simulink model "pfb_fir"  (Simulink 7.0)
settings: Solver=FixedStepDiscrete  SolverMode=SingleTasking  StartTime=0.0  StopTime=10.0  RelTol=1e-3
undefined symbols (not defined in the file): pfb_coefs
libraries: xbsIndex_r4 x385
(part 9 of 27)

== system pfb_fir/fir_2/fir_tap_2 ==
  data_in : Inport  OutDataType=sfix(16)  OutScaling=2^0
  sum_in : Inport  Port=2  OutDataType=sfix(16)  OutScaling=2^0
  sync_in : Inport  Port=3  OutDataType=sfix(16)  OutScaling=2^0
  fir_coef : Subsystem  mask(FIR Filter Coefficient Generator){coef=[-0.000375660323525046;-0.00112528207646786;-0.00187263770065757;-0.00261772609063303;-0.00336054616203061;-0.00410109685156988;-0.00483937711704019;-0.00557538593728603;-0.00630912231219222;-0.00704058526266978;-0.00776977383064064;-0.00849668707902262;-0.00922132409171369;-0.00994368397357705;-0.0106637658504249;-0.0113815688690025;-0.0120970921969721;-0.0128103350228962;-0.0135212965562215;-0.0142299760272615;-0.0149363726871797;-0.0156404858079725;-0.0163423146824514;-0.0170418586242254;-0.0177391169676835;-0.0184340890679761;-0.0191267743009973;-0.0198171720633655;-0.0205052817724058;-0.0211911028661302;-0.0218746348032188;-0.0225558770630009;-0.0232348291454347;-0.0239114905710882;-0.0245858608811188;-0.0252579396372536;-0.0259277264217688;-0.0265952208374693;-0.0272604225076676;-0.0279233310761635;-0.0285839462072226;-0.0292422675855545;-0.0298982949162921;-0.0305520279249694;-0.0312034663574997;-0.031852609980153;-0.0324994585795345;-0.0331440119625613;-0.0337862699564402;-0.0344262324086442;-0.0350638991868898;-0.0356992701791137;-0.0363323452934489;-0.0369631244582015;-0.0375916076218262;-0.0382177947529027;-0.0388416858401109;-0.0394632808922069;-0.0400825799379981;-0.0406995830263182;-0.0413142902260021;-0.0419267016258609;-0.0425368173346564;-0.0431446374810749;-0.0437501622137022;-0.0443533917009969;-0.0449543261312647;-0.0455529657126312;-0.0461493106730163;-0.0467433612601067;-0.047335117741329;-0.0479245804038229;-0.0485117495544134;-0.0490966255195838;-0.0496792086454471;-0.0502594992977191;-0.0508374978616896;-0.0514132047421944;-0.0519866203635867;-0.0525577451697087;-0.0531265796238626;-0.0536931242087811;-0.0542573794265993;-0.0548193457988244;-0.0553790238663066;-0.0559364141892089;-0.0564915173469777;-0.0570443339383125;-0.0575948645811356;-0.0581431099125613;-0.058689070588866;-0.0592327472854569;-0.0597741406968409;-0.0603132515365938;-0.0608500805373288;-0.0613846284506648;-0.0619168960471949;-0.0624468841164546;-0.0629745934668896;-0.0635000249258237;-0.064023179339426;-0.0645440575726791;-0.0650626605093458;-0.0655789890519362;-0.0660930441216749;-0.0666048266584676;-0.0671143376208679;-0.067621577986043;-0.0681265487497408;-0.0686292509262558;-0.0691296855483946;-0.0696278536674418;-0.0701237563531258;-0.0706173946935843;-0.071108769795329;-0.071597882783211;-0.0720847348003859;-0.0725693270082785;-0.0730516605865468;-0.0735317367330474;-0.0740095566637989;-0.0744851216129466;-0.0749584328327259;-0.0754294915934268;-0.0758982991833568;-0.0763648569088048;-0.0768291660940042;-0.0772912280810962;-0.0777510442300928;-0.0782086159188393;-0.0786639445429775;-0.0791170315159078;-0.0795678782687517;-0.0800164862503141;-0.0804628569270452;-0.0809069917830028;-0.0813488923198131;-0.0817885600566336;-0.0822259965301136;-0.0826612032943558;-0.0830941819208773;-0.0835249339985711;-0.0839534611336661;-0.0843797649496887;-0.0848038470874227;-0.0852257092048699;-0.0856453529772106;-0.0860627800967632;-0.0864779922729447;-0.0868909912322302;-0.0873017787181127;-0.0877103564910625;-0.0881167263284868;-0.0885208900246886;-0.0889228493908263;-0.0893226062548723;-0.0897201624615717;-0.0901155198724016;-0.0905086803655288;-0.0908996458357691;-0.0912884181945446;-0.0916749993698427;-0.0920593913061736;-0.0924415959645284;-0.0928216153223364;-0.0931994513734234;-0.0935751061279683;-0.0939485816124612;-0.09431987986966;-0.0946890029585477;-0.0950559529542894;-0.0954207319481889;-0.0957833420476455;-0.0961437853761105;-0.0965020640730433;-0.0968581802938682;-0.0972121362099301;-0.0975639340084509;-0.0979135758924848;-0.0982610640808748;-0.0986064008082076;-0.0989495883247697;-0.0992906288965024;-0.0996295248049575;-0.0999662783472516;-0.100300891836022;-0.100633367599381;-0.100963707980872;-0.101291915339421;-0.101617992049296;-0.101941940500055;-0.102263763096507;-0.102583462258662;-0.102901040421687;-0.103216500035856;-0.103529843566511;-0.103841073494009;-0.104150192313679;-0.104457202535775;-0.104762106685429 ...(+16057 chars)], n_bits_c=9, bin_pt_c=8, use_bram=on}
      mask prompts: coef "Tap Coefficient(s)"; n_bits_c "Number of Coefficient Bits"; bin_pt_c "Coefficient Binary Point"; use_bram "Use BRAM for Coefficients"
      mask help: A Finite Impluse Response filter coefficient generator. This FIR filter coefficient generator outputs real coefficients. It can output one coefficient or cycle through a vector of coefficients for WOLA (Weighted OverLap Add) FIR filters.
      settings: AttributesFormatString=1024 coefs in bram
      mask Help:
      | <pre>
      | Description::
      | 
      | A Finite Impluse Response filter coefficient generator.
      | This FIR filter coefficient generator outputs real coefficients.
      | It can output one coefficient or cycle through a vector of coefficients for WOLA
      | (Weighted OverLap Add) FIR filters.
      | 
      | Mask Parameters::
      | 
      | Tap Coefficiant(s) (coef): The coefficient(s) to output.  For a "regular" FIR filter, this will be a
      | single number.  For a WOLA (Weighted OverLap Add) filter, this will be a vector of numbers.
      | These should be specified as doubles.   They will be rounded and saturated according to the
      | specified number of bits (n_bits_c) and binary point (bin_pt_c).
      | 
      | Number of Coefficient Bits (n_bits_c): The number of bits used for the fixed point binary
      | representation of the coefficient(s).
      | 
      | Coefficient Binary Point (bin_pt_c): The binary point of the fixed point binary representation
      | of the coefficient(s).
      | 
      | Use BRAM for Coefficients (use_bram): Check this checkbox to store the coefficients in BRAM.
      | If unchecked, the coefficients will be stored in distributed memory (i.e. slices).
      | This is only relevant is length(coef) is greater than 1; otherwise, a constant block is used.
      | </pre>
  fir_core : Subsystem  mask(FIR Filter Core){delay=1024, n_bits_d=8, bin_pt_d=7, n_bits_s=17, bin_pt_s=15, use_bram=on, mult_latency=3, add_latency=1, add_bypass=off}
      mask prompts: delay "Tap Delay"; n_bits_d "Number of Data Bits"; bin_pt_d "Data Binary Point"; n_bits_s "Number of Sum Bits"; bin_pt_s "Sum Binary Point"; use_bram "Use BRAM for Delay"; mult_latency "Multiplier Latency"; add_latency "Adder Latency"; add_bypass "Bypass Adder"
      mask help: A Finite Impluse Response Filter core with complex inputs and real coefficients. This FIR filter core does not have provisions for folding the input sequence to improve multiplier efficiency, so it is suboptimal for "regular" (i.e. non-WOLA) FIR filters. It is intended primarily for WOLA (Weighted OverLap Add) FIR filters.
      settings: AttributesFormatString=delay 1024 in bram
      mask Help:
      | <pre>
      | Description::
      | 
      | A Finite Impluse Response Filter core with complex inputs and real coefficients.
      | 
      | This Finite Impluse Response Filter core is designed to be paired with a FIR Coefficient Generator
      | to form a FIR filter tap.  This FIR filter core does not have provisions for folding the input
      | sequence to improve multiplier efficiency, so it is suboptimal for "regular" (i.e. non-WOLA)
      | FIR filters.  It is intended primarily for WOLA (Weighted OverLap Add) FIR filters.
      | 
      | Mask Parameters::
      | 
      | Tap Delay (delay):  The inter-tap delay (the N in "z^-N").  For a regular FIR filter, this will be 1.
      | 
      | Number of Data Bits (n_bits_d): The number of bits for real/imaginary components of the data.
      | 
      | Data Binary Point (bin_pt_d): The binary point for real/imaginary components of the data.
      | 
      | Number of Sum Bits (n_bits_s): Specifies the width of the sum (overflow wraps).
      | 
      | Sum Binary Point (bin_pt_s): Specifies the binary point of the sum (quantization truncates).
      | 
      | Use BRAM for Delay (use_bram): Check this checkbox to implement the delay using BRAM.
      | If unchecked, the delay will be implemented using SLR16 elements (i.e. slices).
      | 
      | Multiplier Latency (mult_latency): Latency to use for the underlying multiplier.
      | 
      | Adder Latency (add_latency): Latency to use for the underlying adder.
      | 
      | Adder Bypass (add_bypass): Check this checkbox to bypass the adder.
      | Typically used for the first tap of a multi-tap FIR filter.
      | </pre>
  data_out : Outport  OutDataType=sfix(16)  OutScaling=2^0
  sum_out : Outport  Port=2  OutDataType=sfix(16)  OutScaling=2^0
  sync_out : Outport  Port=3  OutDataType=sfix(16)  OutScaling=2^0
  wires:
  fir_core/3(sync_out) -> sync_out/1
  fir_core/2(sum_out) -> sum_out/1
  fir_core/1(data_out) -> data_out/1
  sync_in/1 -> fir_coef/3(sync_in)
  sum_in/1 -> fir_coef/2(sum_in)
  data_in/1 -> fir_coef/1(data_in)
  fir_coef/4(sync_out) -> fir_core/4(sync_in)
  fir_coef/3(coef) -> fir_core/3(coef)
  fir_coef/2(sum_out) -> fir_core/2(sum_in)
  fir_coef/1(data_out) -> fir_core/1(data_in)

== system pfb_fir/fir_2/fir_tap_3 ==
  data_in : Inport  OutDataType=sfix(16)  OutScaling=2^0
  sum_in : Inport  Port=2  OutDataType=sfix(16)  OutScaling=2^0
  sync_in : Inport  Port=3  OutDataType=sfix(16)  OutScaling=2^0
  fir_coef : Subsystem  mask(FIR Filter Coefficient Generator){coef=[0.999999547662946;0.999995928971626;0.999988691616268;0.999977835651433;0.999963361158965;0.999945268247983;0.999923557054889;0.99989822774336;0.999869280504348;0.999836715556079;0.999800533144051;0.99976073354103;0.999717317047049;0.999670283989403;0.999619634722648;0.999565369628596;0.999507489116311;0.999445993622108;0.999380883609544;0.999312159569415;0.999239822019754;0.999163871505822;0.999084308600105;0.999001133902306;0.998914348039344;0.998823951665339;0.998729945461616;0.99863233013669;0.998531106426262;0.998426275093213;0.998317836927595;0.998205792746621;0.998090143394661;0.997970889743233;0.99784803269099;0.997721573163716;0.997591512114315;0.997457850522799;0.997320589396285;0.997179729768976;0.997035272702159;0.99688721928419;0.996735570630482;0.996580327883498;0.996421492212737;0.996259064814724;0.996093046912996;0.99592343975809;0.995750244627533;0.995573462825828;0.99539309568444;0.995209144561783;0.995021610843209;0.994830495940991;0.99463580129431;0.994437528369243;0.994235678658745;0.994030253682635;0.993821254987582;0.993608684147091;0.993392542761483;0.993172832457882;0.992949554890201;0.99272271173912;0.992492304712073;0.992258335543232;0.992020805993488;0.991779717850431;0.991535072928337;0.991286873068149;0.991035120137455;0.990779816030475;0.990520962668036;0.990258561997559;0.989992615993036;0.989723126655011;0.989450096010561;0.989173526113274;0.988893419043231;0.988609776906985;0.988322601837537;0.98803189599432;0.987737661563173;0.987439900756322;0.987138615812356;0.986833808996206;0.986525482599124;0.986213638938657;0.985898280358627;0.985579409229105;0.98525702794639;0.984931138932984;0.984601744637569;0.984268847534979;0.98393245012618;0.983592554938246;0.983249164524326;0.98290228146363;0.982551908361392;0.982198047848854;0.981840702583234;0.9814798752477;0.981115568551347;0.980747785229165;0.980376528042017;0.98000179977661;0.979623603245462;0.979241941286885;0.978856816764947;0.978468232569446;0.978076191615887;0.977680696845445;0.977281751224942;0.976879357746813;0.97647351942908;0.976064239315321;0.975651520474639;0.975235366001631;0.97481577901636;0.974392762664321;0.973966320116415;0.973536454568909;0.973103169243412;0.972666467386842;0.972226352271389;0.971782827194488;0.971335895478783;0.970885560472097;0.970431825547395;0.969974694102756;0.969514169561332;0.969050255371323;0.968582955005935;0.96811227196335;0.967638209766689;0.967160771963981;0.966679962128122;0.966195783856846;0.965708240772684;0.965217336522932;0.964723074779614;0.964225459239442;0.963724493623787;0.963220181678634;0.962712527174551;0.962201533906649;0.961687205694544;0.961169546382321;0.960648559838497;0.960124249955978;0.959596620652025;0.959065675868214;0.958531419570396;0.95799385574866;0.957452988417292;0.956908821614734;0.956361359403548;0.955810605870372;0.955256565125884;0.954699241304754;0.954138638565613;0.953574761091004;0.953007613087343;0.952437198784881;0.951863522437655;0.951286588323455;0.950706400743774;0.950122964023769;0.949536282512219;0.948946360581481;0.948353202627446;0.947756813069498;0.947157196350468;0.946554356936591;0.945948299317464;0.945339028005997;0.944726547538374;0.944110862474005;0.943491977395482;0.942869896908532;0.942244625641977;0.941616168247679;0.940984529400506;0.940349713798277;0.939711726161716;0.939070571234412;0.938426253782768;0.937778778595951;0.937128150485851;0.936474374287031;0.935817454856679;0.935157397074559;0.934494205842967;0.933827886086677;0.933158442752899;0.932485880811225;0.931810205253583;0.931131421094187;0.930449533369489;0.929764547138127;0.929076467480875;0.928385299500598;0.927691048322198;0.92699371909256;0.926293316980511;0.925589847176761;0.924883314893854;0.924173725366119;0.923461083849616;0.922745395622088;0.922026665982904;0.92130490025301;0.920580103774877;0.919852281912448;0.919121440051086;0.918387583597519;0.91765071797979;0.9169108486472;0.916167981070258;0.915422120740627;0.914673273171068;0.913921443895387;0.913166638468382 ...(+14460 chars)], n_bits_c=9, bin_pt_c=8, use_bram=on}
      mask prompts: coef "Tap Coefficient(s)"; n_bits_c "Number of Coefficient Bits"; bin_pt_c "Coefficient Binary Point"; use_bram "Use BRAM for Coefficients"
      mask help: A Finite Impluse Response filter coefficient generator. This FIR filter coefficient generator outputs real coefficients. It can output one coefficient or cycle through a vector of coefficients for WOLA (Weighted OverLap Add) FIR filters.
      settings: AttributesFormatString=1024 coefs in bram
      mask Help:
      | <pre>
      | Description::
      | 
      | A Finite Impluse Response filter coefficient generator.
      | This FIR filter coefficient generator outputs real coefficients.
      | It can output one coefficient or cycle through a vector of coefficients for WOLA
      | (Weighted OverLap Add) FIR filters.
      | 
      | Mask Parameters::
      | 
      | Tap Coefficiant(s) (coef): The coefficient(s) to output.  For a "regular" FIR filter, this will be a
      | single number.  For a WOLA (Weighted OverLap Add) filter, this will be a vector of numbers.
      | These should be specified as doubles.   They will be rounded and saturated according to the
      | specified number of bits (n_bits_c) and binary point (bin_pt_c).
      | 
      | Number of Coefficient Bits (n_bits_c): The number of bits used for the fixed point binary
      | representation of the coefficient(s).
      | 
      | Coefficient Binary Point (bin_pt_c): The binary point of the fixed point binary representation
      | of the coefficient(s).
      | 
      | Use BRAM for Coefficients (use_bram): Check this checkbox to store the coefficients in BRAM.
      | If unchecked, the coefficients will be stored in distributed memory (i.e. slices).
      | This is only relevant is length(coef) is greater than 1; otherwise, a constant block is used.
      | </pre>
  fir_core : Subsystem  mask(FIR Filter Core){delay=1024, n_bits_d=8, bin_pt_d=7, n_bits_s=17, bin_pt_s=15, use_bram=on, mult_latency=3, add_latency=1, add_bypass=off}
      mask prompts: delay "Tap Delay"; n_bits_d "Number of Data Bits"; bin_pt_d "Data Binary Point"; n_bits_s "Number of Sum Bits"; bin_pt_s "Sum Binary Point"; use_bram "Use BRAM for Delay"; mult_latency "Multiplier Latency"; add_latency "Adder Latency"; add_bypass "Bypass Adder"
      mask help: A Finite Impluse Response Filter core with complex inputs and real coefficients. This FIR filter core does not have provisions for folding the input sequence to improve multiplier efficiency, so it is suboptimal for "regular" (i.e. non-WOLA) FIR filters. It is intended primarily for WOLA (Weighted OverLap Add) FIR filters.
      settings: AttributesFormatString=delay 1024 in bram
      mask Help:
      | <pre>
      | Description::
      | 
      | A Finite Impluse Response Filter core with complex inputs and real coefficients.
      | 
      | This Finite Impluse Response Filter core is designed to be paired with a FIR Coefficient Generator
      | to form a FIR filter tap.  This FIR filter core does not have provisions for folding the input
      | sequence to improve multiplier efficiency, so it is suboptimal for "regular" (i.e. non-WOLA)
      | FIR filters.  It is intended primarily for WOLA (Weighted OverLap Add) FIR filters.
      | 
      | Mask Parameters::
      | 
      | Tap Delay (delay):  The inter-tap delay (the N in "z^-N").  For a regular FIR filter, this will be 1.
      | 
      | Number of Data Bits (n_bits_d): The number of bits for real/imaginary components of the data.
      | 
      | Data Binary Point (bin_pt_d): The binary point for real/imaginary components of the data.
      | 
      | Number of Sum Bits (n_bits_s): Specifies the width of the sum (overflow wraps).
      | 
      | Sum Binary Point (bin_pt_s): Specifies the binary point of the sum (quantization truncates).
      | 
      | Use BRAM for Delay (use_bram): Check this checkbox to implement the delay using BRAM.
      | If unchecked, the delay will be implemented using SLR16 elements (i.e. slices).
      | 
      | Multiplier Latency (mult_latency): Latency to use for the underlying multiplier.
      | 
      | Adder Latency (add_latency): Latency to use for the underlying adder.
      | 
      | Adder Bypass (add_bypass): Check this checkbox to bypass the adder.
      | Typically used for the first tap of a multi-tap FIR filter.
      | </pre>
  data_out : Outport  OutDataType=sfix(16)  OutScaling=2^0
  sum_out : Outport  Port=2  OutDataType=sfix(16)  OutScaling=2^0
  sync_out : Outport  Port=3  OutDataType=sfix(16)  OutScaling=2^0
  wires:
  fir_core/3(sync_out) -> sync_out/1
  fir_core/2(sum_out) -> sum_out/1
  fir_core/1(data_out) -> data_out/1
  sync_in/1 -> fir_coef/3(sync_in)
  sum_in/1 -> fir_coef/2(sum_in)
  data_in/1 -> fir_coef/1(data_in)
  fir_coef/4(sync_out) -> fir_core/4(sync_in)
  fir_coef/3(coef) -> fir_core/3(coef)
  fir_coef/2(sum_out) -> fir_core/2(sum_in)
  fir_coef/1(data_out) -> fir_core/1(data_in)
